simulink model "sf_sawtooth2_2018a"  (R2018a)
settings: Solver=VariableStepAuto  StartTime=0.0  StopTime=10.0  RelTol=1e-3
settings Model: Creator=bzhan  LastModifiedBy=bzhan
settings DataIOCC: ReturnWorkspaceOutputs=on
settings SFSimCC: SimUseLocalCustomCode=on
settings RTWCC: RTWUseLocalCustomCode=on

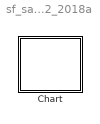
== system sf_sawtooth2_2018a ==
  Chart : Stateflow chart  TreatAsAtomicUnit=on

== stateflow chart sf_sawtooth2_2018a/Chart ==
  settings: updateMethod=CONTINUOUS
  state A
    du: x_dot=1;
  state B
    du: x_dot=-1;
  (default) -> A : {x=0}
  B -> A : [x<=0]
  A -> B : [x>=1]
  data: x local
  data x settings: updateMethod=SF_CONTINUOUS_TIME_DATA
